simulink model "test_p"  (R2022a)
settings: Solver=FixedStepAuto  StartTime=0.0  StopTime=20  FixedStep=0.005  RelTol=1e-3
values from neighbouring files (symbols this model uses):
  AttDyna_Ixx = 0.0211    [InitParameters.m]
  AttDyna_Iyy = 0.0219    [InitParameters.m]
  AttDyna_Izz = 0.0366    [InitParameters.m]
  ConEfficiency_drone_cM = 1.779e-07    [InitParameters.m]
  ConEfficiency_drone_cT = 1.105e-05    [InitParameters.m]
  ConEfficiency_drone_R = 0.225    [InitParameters.m]
  PowerUnit_CR = 1148    [InitParameters.m]
  PowerUnit_Tm = 0.02    [InitParameters.m]
  PowerUnit_wb = -141.4    [InitParameters.m]
libraries: simulink x53, slpidlib x15, fuzblock x12, mpclib x1
(part 3 of 3)

== system test_p/四旋翼模型(简化)1/动力模型 ==
  In1 : Inport
  In2 : Inport  Port=2
  In3 : Inport  Port=3
  In4 : Inport  Port=4
  Constant{,1..3} (4 alike) : Constant  Value=1000
  Gain{,1..3} (4 alike) : Gain  Gain=1/1000
  Motor_Dynamics_1 : StateSpace  Commented=on  A=-1/PowerUnit_Tm  C=1/PowerUnit_Tm  D=0  InitialCondition=557.142*PowerUnit_Tm
  Motor_Dynamics_{2..5} (4 alike) : StateSpace  A=-1/PowerUnit_Tm  C=1/PowerUnit_Tm  D=0  InitialCondition=557.142*PowerUnit_Tm
  Mux : Mux
  Scope{,1..3} (4 alike) : Scope
  Subsystem : Subsystem
  Subsystem1 : Subsystem
  Subsystem2 : Subsystem
  Subsystem3 : Subsystem
  Sum{,1..3} (4 alike) : Sum  Inputs=|+-
  Transfer Fcn5 : TransferFcn  Commented=on  Denominator=[PowerUnit_Tm 1]
  Out1 : Outport  VectorParamsAs1DForOutWhenUnconnected=off
  wires:
  Subsystem2/1(Wss) -> Motor_Dynamics_4/1
  Mux/1 -> Out1/1
  Subsystem1/1(Wss) -> Motor_Dynamics_3/1
  Subsystem3/1(Wss) -> Motor_Dynamics_5/1
  Motor_Dynamics_2/1 -> Mux/1
  Motor_Dynamics_4/1 -> Mux/3
  Subsystem/1(Wss) -> Motor_Dynamics_2/1
  Motor_Dynamics_3/1 -> Mux/2
  Motor_Dynamics_5/1 -> Mux/4
  In1/1 -> Sum/1
  Sum/1 -> Scope3/1, Gain/1
  Gain/1 -> Subsystem/1("throttle_cmd ")
  Constant/1 -> Sum/2
  Constant1/1 -> Sum1/2
  Sum1/1 -> Scope2/1, Gain1/1
  In2/1 -> Sum1/1
  Gain1/1 -> Subsystem1/1("throttle_cmd ")
  In3/1 -> Sum2/1
  Sum2/1 -> Scope1/1, Gain2/1
  Constant2/1 -> Sum2/2
  Gain2/1 -> Subsystem2/1("throttle_cmd ")
  Constant3/1 -> Sum3/2
  Sum3/1 -> Scope/1, Gain3/1
  In4/1 -> Sum3/1
  Gain3/1 -> Subsystem3/1("throttle_cmd ")

== system test_p/四旋翼模型(简化)1/姿态动力学 ==
  note: Subsystem2
  t_x : Inport
  t_y : Inport  Port=2
  t_z : Inport  Port=3
  Constant1 : Constant  Value=AttDyna_Ixx
  Constant2 : Constant  Value=AttDyna_Izz
  Constant4 : Constant  Value=AttDyna_Iyy
  Integrator6 : Integrator
  Integrator7 : Integrator
  Integrator8 : Integrator
  Mux : Mux  Inputs=3
  att_dyna : MATLAB Function  TreatAsAtomicUnit=on
  wb_vector : Outport  VectorParamsAs1DForOutWhenUnconnected=off
  wbx : Outport  Port=2  VectorParamsAs1DForOutWhenUnconnected=off
  wby : Outport  Port=3  VectorParamsAs1DForOutWhenUnconnected=off
  wbz : Outport  Port=4  VectorParamsAs1DForOutWhenUnconnected=off
  wires:
  att_dyna/3(wbz_d) -> Integrator8/1
  att_dyna/2(wby_d) -> Integrator7/1
  att_dyna/1(wbx_d) -> Integrator6/1
  t_y/1 -> att_dyna/5(t_y)
  t_z/1 -> att_dyna/6(t_z)
  t_x/1 -> att_dyna/4(t_x)
  Integrator8/1 -> Mux/3, wbz/1
  Integrator6/1 -> Mux/1, wbx/1
  Integrator7/1 -> Mux/2, wby/1
  Constant2/1 -> att_dyna/3(Izz)
  Constant4/1 -> att_dyna/2(Iyy)
  Constant1/1 -> att_dyna/1(Ixx)
  Mux/1 -> wb_vector/1

== system test_p/四旋翼模型(简化)1/姿态运动学 ==
  pitch : Inport
  roll : Inport  Port=2
  wbx : Inport  Port=3
  wby : Inport  Port=4
  wbz : Inport  Port=5
  Integrator10 : Integrator
  Integrator11 : Integrator
  Integrator9 : Integrator
  att_kine : MATLAB Function  TreatAsAtomicUnit=on
  pitch_ : Outport  VectorParamsAs1DForOutWhenUnconnected=off
  roll_ : Outport  Port=2  VectorParamsAs1DForOutWhenUnconnected=off
  yaw : Outport  Port=3  VectorParamsAs1DForOutWhenUnconnected=off
  wires:
  Integrator9/1 -> roll_/1
  att_kine/1(roll_dot) -> Integrator9/1
  att_kine/2(pitch_dot) -> Integrator10/1
  Integrator11/1 -> yaw/1
  Integrator10/1 -> pitch_/1
  att_kine/3(yaw_dot) -> Integrator11/1
  roll/1 -> att_kine/5(roll)
  pitch/1 -> att_kine/4(pitch)
  wbx/1 -> att_kine/1(wbx)
  wby/1 -> att_kine/2(wby)
  wbz/1 -> att_kine/3(wbz)

== system test_p/四旋翼模型(简化)1/控制效率模型 ==
  w1 : Inport
  w2 : Inport  Port=2
  w3 : Inport  Port=3
  w4 : Inport  Port=4
  Constant5 : Constant  Value=ConEfficiency_drone_R
  Constant6 : Constant  Value=ConEfficiency_drone_cT
  Constant8 : Constant  Value=ConEfficiency_drone_cM
  control_efficiency : MATLAB Function  TreatAsAtomicUnit=on
  f : Outport  VectorParamsAs1DForOutWhenUnconnected=off
  t_x : Outport  Port=2  VectorParamsAs1DForOutWhenUnconnected=off
  t_y : Outport  Port=3  VectorParamsAs1DForOutWhenUnconnected=off
  t_z : Outport  Port=4  VectorParamsAs1DForOutWhenUnconnected=off
  wires:
  control_efficiency/1(f) -> f/1
  control_efficiency/4(t_z) -> t_z/1
  w4/1 -> control_efficiency/4(w4)
  control_efficiency/2(t_x) -> t_x/1
  w3/1 -> control_efficiency/3(w3)
  control_efficiency/3(t_y) -> t_y/1
  w2/1 -> control_efficiency/2(w2)
  Constant8/1 -> control_efficiency/7(cm)
  w1/1 -> control_efficiency/1(w1)
  Constant5/1 -> control_efficiency/5(d)
  Constant6/1 -> control_efficiency/6(ct)

== system test_p/四旋翼模型(简化)2/Control efficiency model ==
  w1 : Inport
  w2 : Inport  Port=2
  w3 : Inport  Port=3
  w4 : Inport  Port=4
  Constant5 : Constant  Value=ConEfficiency_drone_R
  Constant6 : Constant  Value=ConEfficiency_drone_cT
  Constant8 : Constant  Value=ConEfficiency_drone_cM
  control_efficiency : MATLAB Function  TreatAsAtomicUnit=on
  f : Outport  VectorParamsAs1DForOutWhenUnconnected=off
  t_x : Outport  Port=2  VectorParamsAs1DForOutWhenUnconnected=off
  t_y : Outport  Port=3  VectorParamsAs1DForOutWhenUnconnected=off
  t_z : Outport  Port=4  VectorParamsAs1DForOutWhenUnconnected=off
  wires:
  control_efficiency/1(f) -> f/1
  control_efficiency/4(t_z) -> t_z/1
  w4/1 -> control_efficiency/4(w4)
  control_efficiency/2(t_x) -> t_x/1
  w3/1 -> control_efficiency/3(w3)
  control_efficiency/3(t_y) -> t_y/1
  w2/1 -> control_efficiency/2(w2)
  Constant8/1 -> control_efficiency/7(cm)
  w1/1 -> control_efficiency/1(w1)
  Constant5/1 -> control_efficiency/5(d)
  Constant6/1 -> control_efficiency/6(ct)

== system test_p/四旋翼模型(简化)2/Kinetic model ==
  In1 : Inport
  In2 : Inport  Port=2
  In3 : Inport  Port=3
  In4 : Inport  Port=4
  Constant{,1..3} (4 alike) : Constant  Value=1000
  Gain{,1..3} (4 alike) : Gain  Gain=1/1000
  Motor_Dynamics_1 : StateSpace  Commented=on  A=-1/PowerUnit_Tm  C=1/PowerUnit_Tm  D=0  InitialCondition=557.142*PowerUnit_Tm
  Motor_Dynamics_{2..5} (4 alike) : StateSpace  A=-1/PowerUnit_Tm  C=1/PowerUnit_Tm  D=0  InitialCondition=557.142*PowerUnit_Tm
  Mux : Mux
  Scope{,1..3} (4 alike) : Scope
  Subsystem : Subsystem
  Subsystem1 : Subsystem
  Subsystem2 : Subsystem
  Subsystem3 : Subsystem
  Sum{,1..3} (4 alike) : Sum  Inputs=|+-
  Transfer Fcn5 : TransferFcn  Commented=on  Denominator=[PowerUnit_Tm 1]
  Out1 : Outport  VectorParamsAs1DForOutWhenUnconnected=off
  wires:
  Subsystem2/1(Wss) -> Motor_Dynamics_4/1
  Mux/1 -> Out1/1
  Subsystem1/1(Wss) -> Motor_Dynamics_3/1
  Subsystem3/1(Wss) -> Motor_Dynamics_5/1
  Motor_Dynamics_2/1 -> Mux/1
  Motor_Dynamics_4/1 -> Mux/3
  Subsystem/1(Wss) -> Motor_Dynamics_2/1
  Motor_Dynamics_3/1 -> Mux/2
  Motor_Dynamics_5/1 -> Mux/4
  In1/1 -> Sum/1
  Sum/1 -> Scope3/1, Gain/1
  Gain/1 -> Subsystem/1("throttle_cmd ")
  Constant/1 -> Sum/2
  Constant1/1 -> Sum1/2
  Sum1/1 -> Scope2/1, Gain1/1
  In2/1 -> Sum1/1
  Gain1/1 -> Subsystem1/1("throttle_cmd ")
  In3/1 -> Sum2/1
  Sum2/1 -> Scope1/1, Gain2/1
  Constant2/1 -> Sum2/2
  Gain2/1 -> Subsystem2/1("throttle_cmd ")
  Constant3/1 -> Sum3/2
  Sum3/1 -> Scope/1, Gain3/1
  In4/1 -> Sum3/1
  Gain3/1 -> Subsystem3/1("throttle_cmd ")

== system test_p/四旋翼模型(简化)2/Posture Kinematics ==
  pitch : Inport
  roll : Inport  Port=2
  wbx : Inport  Port=3
  wby : Inport  Port=4
  wbz : Inport  Port=5
  Integrator10 : Integrator
  Integrator11 : Integrator
  Integrator9 : Integrator
  att_kine : MATLAB Function  TreatAsAtomicUnit=on
  pitch_ : Outport  VectorParamsAs1DForOutWhenUnconnected=off
  roll_ : Outport  Port=2  VectorParamsAs1DForOutWhenUnconnected=off
  yaw : Outport  Port=3  VectorParamsAs1DForOutWhenUnconnected=off
  wires:
  Integrator9/1 -> roll_/1
  att_kine/1(roll_dot) -> Integrator9/1
  att_kine/2(pitch_dot) -> Integrator10/1
  Integrator11/1 -> yaw/1
  Integrator10/1 -> pitch_/1
  att_kine/3(yaw_dot) -> Integrator11/1
  roll/1 -> att_kine/5(roll)
  pitch/1 -> att_kine/4(pitch)
  wbx/1 -> att_kine/1(wbx)
  wby/1 -> att_kine/2(wby)
  wbz/1 -> att_kine/3(wbz)

== system test_p/四旋翼模型(简化)2/Posture dynamics ==
  note: Subsystem2
  t_x : Inport
  t_y : Inport  Port=2
  t_z : Inport  Port=3
  Constant1 : Constant  Value=AttDyna_Ixx
  Constant2 : Constant  Value=AttDyna_Izz
  Constant4 : Constant  Value=AttDyna_Iyy
  Integrator6 : Integrator
  Integrator7 : Integrator
  Integrator8 : Integrator
  Mux : Mux  Inputs=3
  att_dyna : MATLAB Function  TreatAsAtomicUnit=on
  wb_vector : Outport  VectorParamsAs1DForOutWhenUnconnected=off
  wbx : Outport  Port=2  VectorParamsAs1DForOutWhenUnconnected=off
  wby : Outport  Port=3  VectorParamsAs1DForOutWhenUnconnected=off
  wbz : Outport  Port=4  VectorParamsAs1DForOutWhenUnconnected=off
  wires:
  att_dyna/3(wbz_d) -> Integrator8/1
  att_dyna/2(wby_d) -> Integrator7/1
  att_dyna/1(wbx_d) -> Integrator6/1
  t_y/1 -> att_dyna/5(t_y)
  t_z/1 -> att_dyna/6(t_z)
  t_x/1 -> att_dyna/4(t_x)
  Integrator8/1 -> Mux/3, wbz/1
  Integrator6/1 -> Mux/1, wbx/1
  Integrator7/1 -> Mux/2, wby/1
  Constant2/1 -> att_dyna/3(Izz)
  Constant4/1 -> att_dyna/2(Iyy)
  Constant1/1 -> att_dyna/1(Ixx)
  Mux/1 -> wb_vector/1

== system test_p/四旋翼模型(简化)3/动力模型 ==
  In1 : Inport
  In2 : Inport  Port=2
  In3 : Inport  Port=3
  In4 : Inport  Port=4
  Constant{,1..3} (4 alike) : Constant  Value=1000
  Gain{,1..3} (4 alike) : Gain  Gain=1/1000
  Motor_Dynamics_1 : StateSpace  Commented=on  A=-1/PowerUnit_Tm  C=1/PowerUnit_Tm  D=0  InitialCondition=557.142*PowerUnit_Tm
  Motor_Dynamics_{2..5} (4 alike) : StateSpace  A=-1/PowerUnit_Tm  C=1/PowerUnit_Tm  D=0  InitialCondition=557.142*PowerUnit_Tm
  Mux : Mux
  Scope{,1..3} (4 alike) : Scope
  Subsystem : Subsystem
  Subsystem1 : Subsystem
  Subsystem2 : Subsystem
  Subsystem3 : Subsystem
  Sum{,1..3} (4 alike) : Sum  Inputs=|+-
  Transfer Fcn5 : TransferFcn  Commented=on  Denominator=[PowerUnit_Tm 1]
  Out1 : Outport  VectorParamsAs1DForOutWhenUnconnected=off
  wires:
  Subsystem2/1(Wss) -> Motor_Dynamics_4/1
  Mux/1 -> Out1/1
  Subsystem1/1(Wss) -> Motor_Dynamics_3/1
  Subsystem3/1(Wss) -> Motor_Dynamics_5/1
  Motor_Dynamics_2/1 -> Mux/1
  Motor_Dynamics_4/1 -> Mux/3
  Subsystem/1(Wss) -> Motor_Dynamics_2/1
  Motor_Dynamics_3/1 -> Mux/2
  Motor_Dynamics_5/1 -> Mux/4
  In1/1 -> Sum/1
  Sum/1 -> Scope3/1, Gain/1
  Gain/1 -> Subsystem/1("throttle_cmd ")
  Constant/1 -> Sum/2
  Constant1/1 -> Sum1/2
  Sum1/1 -> Scope2/1, Gain1/1
  In2/1 -> Sum1/1
  Gain1/1 -> Subsystem1/1("throttle_cmd ")
  In3/1 -> Sum2/1
  Sum2/1 -> Scope1/1, Gain2/1
  Constant2/1 -> Sum2/2
  Gain2/1 -> Subsystem2/1("throttle_cmd ")
  Constant3/1 -> Sum3/2
  Sum3/1 -> Scope/1, Gain3/1
  In4/1 -> Sum3/1
  Gain3/1 -> Subsystem3/1("throttle_cmd ")

== system test_p/四旋翼模型(简化)3/姿态动力学 ==
  note: Subsystem2
  t_x : Inport
  t_y : Inport  Port=2
  t_z : Inport  Port=3
  Constant1 : Constant  Value=AttDyna_Ixx
  Constant2 : Constant  Value=AttDyna_Izz
  Constant4 : Constant  Value=AttDyna_Iyy
  Integrator6 : Integrator
  Integrator7 : Integrator
  Integrator8 : Integrator
  Mux : Mux  Inputs=3
  att_dyna : MATLAB Function  TreatAsAtomicUnit=on
  wb_vector : Outport  VectorParamsAs1DForOutWhenUnconnected=off
  wbx : Outport  Port=2  VectorParamsAs1DForOutWhenUnconnected=off
  wby : Outport  Port=3  VectorParamsAs1DForOutWhenUnconnected=off
  wbz : Outport  Port=4  VectorParamsAs1DForOutWhenUnconnected=off
  wires:
  att_dyna/3(wbz_d) -> Integrator8/1
  att_dyna/2(wby_d) -> Integrator7/1
  att_dyna/1(wbx_d) -> Integrator6/1
  t_y/1 -> att_dyna/5(t_y)
  t_z/1 -> att_dyna/6(t_z)
  t_x/1 -> att_dyna/4(t_x)
  Integrator8/1 -> Mux/3, wbz/1
  Integrator6/1 -> Mux/1, wbx/1
  Integrator7/1 -> Mux/2, wby/1
  Constant2/1 -> att_dyna/3(Izz)
  Constant4/1 -> att_dyna/2(Iyy)
  Constant1/1 -> att_dyna/1(Ixx)
  Mux/1 -> wb_vector/1

== system test_p/四旋翼模型(简化)3/姿态运动学 ==
  pitch : Inport
  roll : Inport  Port=2
  wbx : Inport  Port=3
  wby : Inport  Port=4
  wbz : Inport  Port=5
  Integrator10 : Integrator
  Integrator11 : Integrator
  Integrator9 : Integrator
  att_kine : MATLAB Function  TreatAsAtomicUnit=on
  pitch_ : Outport  VectorParamsAs1DForOutWhenUnconnected=off
  roll_ : Outport  Port=2  VectorParamsAs1DForOutWhenUnconnected=off
  yaw : Outport  Port=3  VectorParamsAs1DForOutWhenUnconnected=off
  wires:
  Integrator9/1 -> roll_/1
  att_kine/1(roll_dot) -> Integrator9/1
  att_kine/2(pitch_dot) -> Integrator10/1
  Integrator11/1 -> yaw/1
  Integrator10/1 -> pitch_/1
  att_kine/3(yaw_dot) -> Integrator11/1
  roll/1 -> att_kine/5(roll)
  pitch/1 -> att_kine/4(pitch)
  wbx/1 -> att_kine/1(wbx)
  wby/1 -> att_kine/2(wby)
  wbz/1 -> att_kine/3(wbz)

== system test_p/四旋翼模型(简化)3/控制效率模型 ==
  w1 : Inport
  w2 : Inport  Port=2
  w3 : Inport  Port=3
  w4 : Inport  Port=4
  Constant5 : Constant  Value=ConEfficiency_drone_R
  Constant6 : Constant  Value=ConEfficiency_drone_cT
  Constant8 : Constant  Value=ConEfficiency_drone_cM
  control_efficiency : MATLAB Function  TreatAsAtomicUnit=on
  f : Outport  VectorParamsAs1DForOutWhenUnconnected=off
  t_x : Outport  Port=2  VectorParamsAs1DForOutWhenUnconnected=off
  t_y : Outport  Port=3  VectorParamsAs1DForOutWhenUnconnected=off
  t_z : Outport  Port=4  VectorParamsAs1DForOutWhenUnconnected=off
  wires:
  control_efficiency/1(f) -> f/1
  control_efficiency/4(t_z) -> t_z/1
  w4/1 -> control_efficiency/4(w4)
  control_efficiency/2(t_x) -> t_x/1
  w3/1 -> control_efficiency/3(w3)
  control_efficiency/3(t_y) -> t_y/1
  w2/1 -> control_efficiency/2(w2)
  Constant8/1 -> control_efficiency/7(cm)
  w1/1 -> control_efficiency/1(w1)
  Constant5/1 -> control_efficiency/5(d)
  Constant6/1 -> control_efficiency/6(ct)

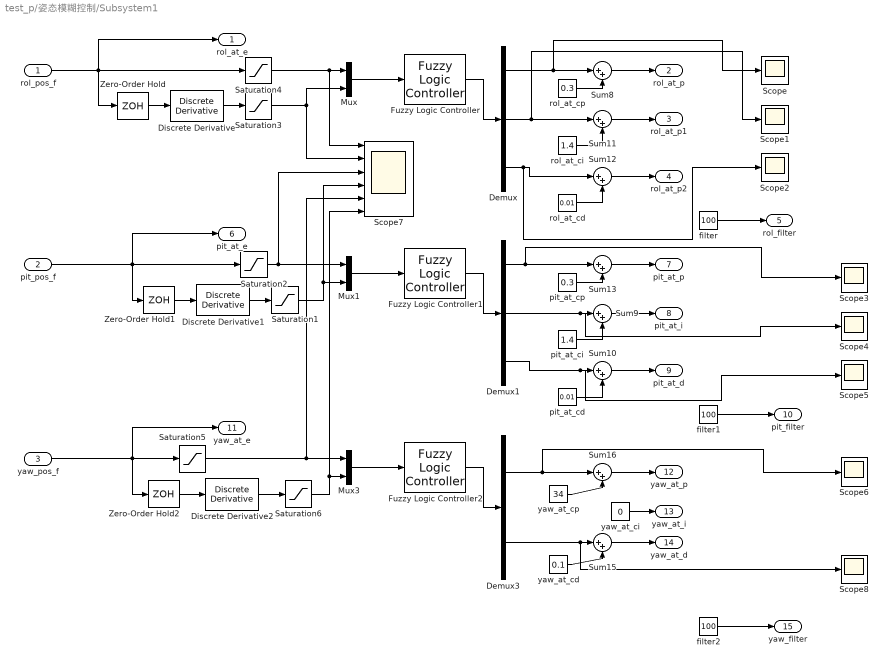
== system test_p/姿态模糊控制/Subsystem1 ==
  rol_pos_f : Inport
  pit_pos_f : Inport  Port=2
  yaw_pos_f : Inport  Port=3
  Demux : Demux  Outputs=3
  Demux1 : Demux  Outputs=3
  Demux3 : Demux  Outputs=2
  Discrete Derivative : simulink/Discrete/Discrete Derivative  gainval=1.0  ICPrevScaledInput=0.0  OutMin=[]  OutMax=[]  OutDataType=fixdt(1, 16)  OutScaling=2^-10  DoSatur=off
  Discrete Derivative1 : simulink/Discrete/Discrete Derivative  gainval=1.0  ICPrevScaledInput=0.0  OutMin=[]  OutMax=[]  OutDataType=fixdt(1, 16)  OutScaling=2^-10  DoSatur=off
  Discrete Derivative2 : simulink/Discrete/Discrete Derivative  gainval=1.0  ICPrevScaledInput=0.0  OutMin=[]  OutMax=[]  OutDataType=fixdt(1, 16)  OutScaling=2^-10  DoSatur=off
  Fuzzy Logic Controller : fuzblock/Fuzzy Logic  Controller  FIS='rol_pit_at.fis'  OutputSampleNumber=101  DataType=double  FuzzifiedInputs=off  RuleFiringStrengths=off  RuleOutputs=off  AggregatedOutputs=off  SimulateUsing=Interpreted execution  OutOfRangeInputValueMessage=warning  NoRuleFiredMessage=warning  EmptyOutputFuzzySetMessage=warning
  Fuzzy Logic Controller1 : fuzblock/Fuzzy Logic  Controller  FIS='rol_pit_at.fis'  OutputSampleNumber=101  DataType=double  FuzzifiedInputs=off  RuleFiringStrengths=off  RuleOutputs=off  AggregatedOutputs=off  SimulateUsing=Interpreted execution  OutOfRangeInputValueMessage=warning  NoRuleFiredMessage=warning  EmptyOutputFuzzySetMessage=warning
  Fuzzy Logic Controller2 : fuzblock/Fuzzy Logic  Controller  FIS='yaw_at.fis'  OutputSampleNumber=101  DataType=double  FuzzifiedInputs=off  RuleFiringStrengths=off  RuleOutputs=off  AggregatedOutputs=off  SimulateUsing=Interpreted execution  OutOfRangeInputValueMessage=warning  NoRuleFiredMessage=warning  EmptyOutputFuzzySetMessage=warning
  Mux : Mux  Inputs=2
  Mux1 : Mux  Inputs=2
  Mux3 : Mux  Inputs=2
  Saturation{1..6} (6 alike) : Saturate  UpperLimit=10  LowerLimit=-10
  Scope{,1..6,8} (8 alike) : Scope
  Scope7 : Scope  NumInputPorts=6
  Sum{8..13,15..16} (8 alike) : Sum  Inputs=|++
  Zero-Order Hold : ZeroOrderHold  SampleTime=-1
  Zero-Order Hold1 : ZeroOrderHold  SampleTime=-1
  Zero-Order Hold2 : ZeroOrderHold  SampleTime=-1
  filter : Constant  Value=100
  filter1 : Constant  Value=100
  filter2 : Constant  Value=100
  pit_at_cd : Constant  Value=0.01
  pit_at_ci : Constant  Value=1.4
  pit_at_cp : Constant  Value=0.3
  rol_at_cd : Constant  Value=0.01
  rol_at_ci : Constant  Value=1.4
  rol_at_cp : Constant  Value=0.3
  yaw_at_cd : Constant  Value=0.1
  yaw_at_ci : Constant  Value=0
  yaw_at_cp : Constant  Value=34
  rol_at_e : Outport  VectorParamsAs1DForOutWhenUnconnected=off
  rol_at_p : Outport  Port=2  VectorParamsAs1DForOutWhenUnconnected=off
  rol_at_p1 : Outport  Port=3  VectorParamsAs1DForOutWhenUnconnected=off
  rol_at_p2 : Outport  Port=4  VectorParamsAs1DForOutWhenUnconnected=off
  rol_filter : Outport  Port=5  VectorParamsAs1DForOutWhenUnconnected=off
  pit_at_e : Outport  Port=6  VectorParamsAs1DForOutWhenUnconnected=off
  pit_at_p : Outport  Port=7  VectorParamsAs1DForOutWhenUnconnected=off
  pit_at_i : Outport  Port=8  VectorParamsAs1DForOutWhenUnconnected=off
  pit_at_d : Outport  Port=9  VectorParamsAs1DForOutWhenUnconnected=off
  pit_filter : Outport  Port=10  VectorParamsAs1DForOutWhenUnconnected=off
  yaw_at_e : Outport  Port=11  VectorParamsAs1DForOutWhenUnconnected=off
  yaw_at_p : Outport  Port=12  VectorParamsAs1DForOutWhenUnconnected=off
  yaw_at_i : Outport  Port=13  VectorParamsAs1DForOutWhenUnconnected=off
  yaw_at_d : Outport  Port=14  VectorParamsAs1DForOutWhenUnconnected=off
  yaw_filter : Outport  Port=15  VectorParamsAs1DForOutWhenUnconnected=off
  wires:
  Discrete Derivative/1 -> Saturation3/1
  rol_at_ci/1 -> Sum11/2
  Mux3/1 -> Fuzzy Logic Controller2/1
  rol_pos_f/1 -> rol_at_e/1, Zero-Order Hold/1, Saturation4/1
  Demux/1 -> Scope/1, Sum8/1
  Zero-Order Hold2/1 -> Discrete Derivative2/1
  Sum12/1 -> rol_at_p2/1
  Demux1/2 -> Scope4/1, Sum9/1
  yaw_at_cp/1 -> Sum16/2
  yaw_pos_f/1 -> yaw_at_e/1, Zero-Order Hold2/1, Saturation5/1
  Sum11/1 -> rol_at_p1/1
  Discrete Derivative2/1 -> Saturation6/1
  Sum9/1 -> pit_at_i/1
  Mux1/1 -> Fuzzy Logic Controller1/1
  Sum13/1 -> pit_at_p/1
  Demux/3 -> Scope2/1, Sum12/1
  Sum8/1 -> rol_at_p/1
  Demux1/1 -> Scope3/1, Sum13/1
  yaw_at_cd/1 -> Sum15/2
  Zero-Order Hold1/1 -> Discrete Derivative1/1
  Zero-Order Hold/1 -> Discrete Derivative/1
  Demux3/1 -> Scope6/1, Sum16/1
  rol_at_cp/1 -> Sum8/2
  Fuzzy Logic Controller2/1 -> Demux3/1
  Sum16/1 -> yaw_at_p/1
  Sum15/1 -> yaw_at_d/1
  rol_at_cd/1 -> Sum12/2
  pit_pos_f/1 -> pit_at_e/1, Zero-Order Hold1/1, Saturation2/1
  Fuzzy Logic Controller1/1 -> Demux1/1
  Fuzzy Logic Controller/1 -> Demux/1
  pit_at_cp/1 -> Sum13/2
  Demux/2 -> Scope1/1, Sum11/1
  Mux/1 -> Fuzzy Logic Controller/1
  pit_at_ci/1 -> Sum9/2
  Sum10/1 -> pit_at_d/1
  Demux1/3 -> Scope5/1, Sum10/1
  pit_at_cd/1 -> Sum10/2
  filter/1 -> rol_filter/1
  filter1/1 -> pit_filter/1
  filter2/1 -> yaw_filter/1
  yaw_at_ci/1 -> yaw_at_i/1
  Demux3/2 -> Scope8/1, Sum15/1
  Discrete Derivative1/1 -> Saturation1/1
  Saturation1/1 -> Scope7/4, Mux1/2
  Saturation2/1 -> Scope7/3, Mux1/1
  Saturation3/1 -> Scope7/2, Mux/2
  Saturation4/1 -> Scope7/1, Mux/1
  Saturation5/1 -> Scope7/5, Mux3/1
  Saturation6/1 -> Scope7/6, Mux3/2

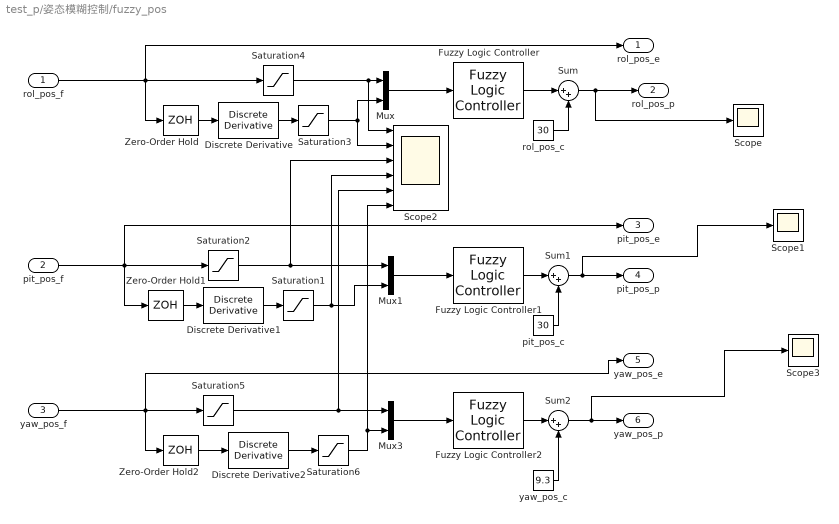
== system test_p/姿态模糊控制/fuzzy_pos ==
  rol_pos_f : Inport
  pit_pos_f : Inport  Port=2
  yaw_pos_f : Inport  Port=3
  Discrete Derivative : simulink/Discrete/Discrete Derivative  gainval=1.0  ICPrevScaledInput=0.0  OutMin=[]  OutMax=[]  OutDataType=fixdt(1, 16)  OutScaling=2^-10  DoSatur=off
  Discrete Derivative1 : simulink/Discrete/Discrete Derivative  gainval=1.0  ICPrevScaledInput=0.0  OutMin=[]  OutMax=[]  OutDataType=fixdt(1, 16)  OutScaling=2^-10  DoSatur=off
  Discrete Derivative2 : simulink/Discrete/Discrete Derivative  gainval=1.0  ICPrevScaledInput=0.0  OutMin=[]  OutMax=[]  OutDataType=fixdt(1, 16)  OutScaling=2^-10  DoSatur=off
  Fuzzy Logic Controller : fuzblock/Fuzzy Logic  Controller  FIS='rol_pit_pos.fis'  OutputSampleNumber=101  DataType=double  FuzzifiedInputs=off  RuleFiringStrengths=off  RuleOutputs=off  AggregatedOutputs=off  SimulateUsing=Interpreted execution  OutOfRangeInputValueMessage=warning  NoRuleFiredMessage=warning  EmptyOutputFuzzySetMessage=warning
  Fuzzy Logic Controller1 : fuzblock/Fuzzy Logic  Controller  FIS='rol_pit_pos.fis'  OutputSampleNumber=101  DataType=double  FuzzifiedInputs=off  RuleFiringStrengths=off  RuleOutputs=off  AggregatedOutputs=off  SimulateUsing=Interpreted execution  OutOfRangeInputValueMessage=warning  NoRuleFiredMessage=warning  EmptyOutputFuzzySetMessage=warning
  Fuzzy Logic Controller2 : fuzblock/Fuzzy Logic  Controller  FIS='yaw_pos.fis'  OutputSampleNumber=101  DataType=double  FuzzifiedInputs=off  RuleFiringStrengths=off  RuleOutputs=off  AggregatedOutputs=off  SimulateUsing=Interpreted execution  OutOfRangeInputValueMessage=warning  NoRuleFiredMessage=warning  EmptyOutputFuzzySetMessage=warning
  Mux : Mux  Inputs=2
  Mux1 : Mux  Inputs=2
  Mux3 : Mux  Inputs=2
  Saturation{1..6} (6 alike) : Saturate  UpperLimit=10  LowerLimit=-10
  Scope : Scope
  Scope1 : Scope
  Scope2 : Scope  NumInputPorts=6
  Scope3 : Scope
  Sum : Sum  Inputs=|++
  Sum1 : Sum  Inputs=|++
  Sum2 : Sum  Inputs=|++
  Zero-Order Hold : ZeroOrderHold  SampleTime=-1
  Zero-Order Hold1 : ZeroOrderHold  SampleTime=-1
  Zero-Order Hold2 : ZeroOrderHold  SampleTime=-1
  pit_pos_c : Constant  Value=30
  rol_pos_c : Constant  Value=30
  yaw_pos_c : Constant  Value=9.3
  rol_pos_e : Outport  VectorParamsAs1DForOutWhenUnconnected=off
  rol_pos_p : Outport  Port=2  VectorParamsAs1DForOutWhenUnconnected=off
  pit_pos_e : Outport  Port=3  VectorParamsAs1DForOutWhenUnconnected=off
  pit_pos_p : Outport  Port=4  VectorParamsAs1DForOutWhenUnconnected=off
  yaw_pos_e : Outport  Port=5  VectorParamsAs1DForOutWhenUnconnected=off
  yaw_pos_p : Outport  Port=6  VectorParamsAs1DForOutWhenUnconnected=off
  wires:
  Zero-Order Hold2/1 -> Discrete Derivative2/1
  pit_pos_f/1 -> pit_pos_e/1, Saturation2/1, Zero-Order Hold1/1
  rol_pos_f/1 -> rol_pos_e/1, Zero-Order Hold/1, Saturation4/1
  yaw_pos_f/1 -> yaw_pos_e/1, Zero-Order Hold2/1, Saturation5/1
  Discrete Derivative/1 -> Saturation3/1
  Mux3/1 -> Fuzzy Logic Controller2/1
  Zero-Order Hold1/1 -> Discrete Derivative1/1
  Mux1/1 -> Fuzzy Logic Controller1/1
  Mux/1 -> Fuzzy Logic Controller/1
  Zero-Order Hold/1 -> Discrete Derivative/1
  Discrete Derivative2/1 -> Saturation6/1
  Fuzzy Logic Controller/1 -> Sum/1
  Sum/1 -> Scope/1, rol_pos_p/1
  rol_pos_c/1 -> Sum/2
  Fuzzy Logic Controller1/1 -> Sum1/1
  pit_pos_c/1 -> Sum1/2
  Sum1/1 -> Scope1/1, pit_pos_p/1
  Fuzzy Logic Controller2/1 -> Sum2/1
  Sum2/1 -> Scope3/1, yaw_pos_p/1
  yaw_pos_c/1 -> Sum2/2
  Discrete Derivative1/1 -> Saturation1/1
  Saturation1/1 -> Scope2/4, Mux1/2
  Saturation2/1 -> Scope2/3, Mux1/1
  Saturation3/1 -> Mux/2, Scope2/2
  Saturation4/1 -> Scope2/1, Mux/1
  Saturation5/1 -> Scope2/5, Mux3/1
  Saturation6/1 -> Scope2/6, Mux3/2

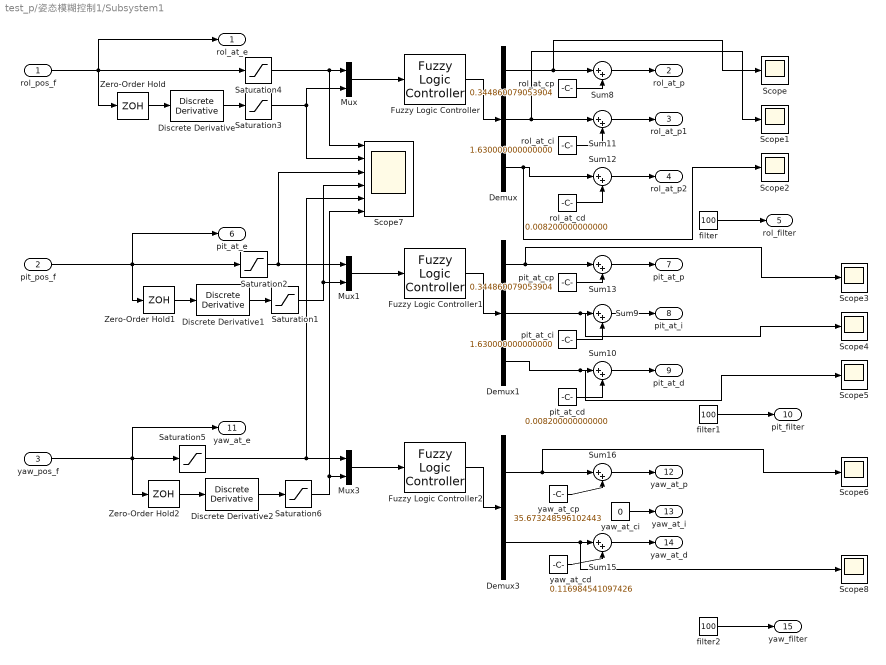
== system test_p/姿态模糊控制1/Subsystem1 ==
  rol_pos_f : Inport
  pit_pos_f : Inport  Port=2
  yaw_pos_f : Inport  Port=3
  Demux : Demux  Outputs=3
  Demux1 : Demux  Outputs=3
  Demux3 : Demux  Outputs=2
  Discrete Derivative : simulink/Discrete/Discrete Derivative  gainval=1.0  ICPrevScaledInput=0.0  OutMin=[]  OutMax=[]  OutDataType=fixdt(1, 16)  OutScaling=2^-10  DoSatur=off
  Discrete Derivative1 : simulink/Discrete/Discrete Derivative  gainval=1.0  ICPrevScaledInput=0.0  OutMin=[]  OutMax=[]  OutDataType=fixdt(1, 16)  OutScaling=2^-10  DoSatur=off
  Discrete Derivative2 : simulink/Discrete/Discrete Derivative  gainval=1.0  ICPrevScaledInput=0.0  OutMin=[]  OutMax=[]  OutDataType=fixdt(1, 16)  OutScaling=2^-10  DoSatur=off
  Fuzzy Logic Controller : fuzblock/Fuzzy Logic  Controller  FIS='rol_pit_at.fis'  OutputSampleNumber=101  DataType=double  FuzzifiedInputs=off  RuleFiringStrengths=off  RuleOutputs=off  AggregatedOutputs=off  SimulateUsing=Interpreted execution  OutOfRangeInputValueMessage=warning  NoRuleFiredMessage=warning  EmptyOutputFuzzySetMessage=warning
  Fuzzy Logic Controller1 : fuzblock/Fuzzy Logic  Controller  FIS='rol_pit_at.fis'  OutputSampleNumber=101  DataType=double  FuzzifiedInputs=off  RuleFiringStrengths=off  RuleOutputs=off  AggregatedOutputs=off  SimulateUsing=Interpreted execution  OutOfRangeInputValueMessage=warning  NoRuleFiredMessage=warning  EmptyOutputFuzzySetMessage=warning
  Fuzzy Logic Controller2 : fuzblock/Fuzzy Logic  Controller  FIS='yaw_at.fis'  OutputSampleNumber=101  DataType=double  FuzzifiedInputs=off  RuleFiringStrengths=off  RuleOutputs=off  AggregatedOutputs=off  SimulateUsing=Interpreted execution  OutOfRangeInputValueMessage=warning  NoRuleFiredMessage=warning  EmptyOutputFuzzySetMessage=warning
  Mux : Mux  Inputs=2
  Mux1 : Mux  Inputs=2
  Mux3 : Mux  Inputs=2
  Saturation{1..6} (6 alike) : Saturate  UpperLimit=10  LowerLimit=-10
  Scope{,1..6,8} (8 alike) : Scope
  Scope7 : Scope  NumInputPorts=6
  Sum{8..13,15..16} (8 alike) : Sum  Inputs=|++
  Zero-Order Hold : ZeroOrderHold  SampleTime=-1
  Zero-Order Hold1 : ZeroOrderHold  SampleTime=-1
  Zero-Order Hold2 : ZeroOrderHold  SampleTime=-1
  filter : Constant  Value=100
  filter1 : Constant  Value=100
  filter2 : Constant  Value=100
  pit_at_cd : Constant  Value=0.008200000000000
  pit_at_ci : Constant  Value=1.630000000000000
  pit_at_cp : Constant  Value=0.344860079053904
  rol_at_cd : Constant  Value=0.008200000000000
  rol_at_ci : Constant  Value=1.630000000000000
  rol_at_cp : Constant  Value=0.344860079053904
  yaw_at_cd : Constant  Value=0.116984541097426
  yaw_at_ci : Constant  Value=0
  yaw_at_cp : Constant  Value=35.673248596102443
  rol_at_e : Outport  VectorParamsAs1DForOutWhenUnconnected=off
  rol_at_p : Outport  Port=2  VectorParamsAs1DForOutWhenUnconnected=off
  rol_at_p1 : Outport  Port=3  VectorParamsAs1DForOutWhenUnconnected=off
  rol_at_p2 : Outport  Port=4  VectorParamsAs1DForOutWhenUnconnected=off
  rol_filter : Outport  Port=5  VectorParamsAs1DForOutWhenUnconnected=off
  pit_at_e : Outport  Port=6  VectorParamsAs1DForOutWhenUnconnected=off
  pit_at_p : Outport  Port=7  VectorParamsAs1DForOutWhenUnconnected=off
  pit_at_i : Outport  Port=8  VectorParamsAs1DForOutWhenUnconnected=off
  pit_at_d : Outport  Port=9  VectorParamsAs1DForOutWhenUnconnected=off
  pit_filter : Outport  Port=10  VectorParamsAs1DForOutWhenUnconnected=off
  yaw_at_e : Outport  Port=11  VectorParamsAs1DForOutWhenUnconnected=off
  yaw_at_p : Outport  Port=12  VectorParamsAs1DForOutWhenUnconnected=off
  yaw_at_i : Outport  Port=13  VectorParamsAs1DForOutWhenUnconnected=off
  yaw_at_d : Outport  Port=14  VectorParamsAs1DForOutWhenUnconnected=off
  yaw_filter : Outport  Port=15  VectorParamsAs1DForOutWhenUnconnected=off
  wires:
  Discrete Derivative/1 -> Saturation3/1
  rol_at_ci/1 -> Sum11/2
  Mux3/1 -> Fuzzy Logic Controller2/1
  rol_pos_f/1 -> rol_at_e/1, Zero-Order Hold/1, Saturation4/1
  Demux/1 -> Scope/1, Sum8/1
  Zero-Order Hold2/1 -> Discrete Derivative2/1
  Sum12/1 -> rol_at_p2/1
  Demux1/2 -> Scope4/1, Sum9/1
  yaw_at_cp/1 -> Sum16/2
  yaw_pos_f/1 -> yaw_at_e/1, Zero-Order Hold2/1, Saturation5/1
  Sum11/1 -> rol_at_p1/1
  Discrete Derivative2/1 -> Saturation6/1
  Sum9/1 -> pit_at_i/1
  Mux1/1 -> Fuzzy Logic Controller1/1
  Sum13/1 -> pit_at_p/1
  Demux/3 -> Scope2/1, Sum12/1
  Sum8/1 -> rol_at_p/1
  Demux1/1 -> Scope3/1, Sum13/1
  yaw_at_cd/1 -> Sum15/2
  Zero-Order Hold1/1 -> Discrete Derivative1/1
  Zero-Order Hold/1 -> Discrete Derivative/1
  Demux3/1 -> Scope6/1, Sum16/1
  rol_at_cp/1 -> Sum8/2
  Fuzzy Logic Controller2/1 -> Demux3/1
  Sum16/1 -> yaw_at_p/1
  Sum15/1 -> yaw_at_d/1
  rol_at_cd/1 -> Sum12/2
  pit_pos_f/1 -> pit_at_e/1, Zero-Order Hold1/1, Saturation2/1
  Fuzzy Logic Controller1/1 -> Demux1/1
  Fuzzy Logic Controller/1 -> Demux/1
  pit_at_cp/1 -> Sum13/2
  Demux/2 -> Scope1/1, Sum11/1
  Mux/1 -> Fuzzy Logic Controller/1
  pit_at_ci/1 -> Sum9/2
  Sum10/1 -> pit_at_d/1
  Demux1/3 -> Scope5/1, Sum10/1
  pit_at_cd/1 -> Sum10/2
  filter/1 -> rol_filter/1
  filter1/1 -> pit_filter/1
  filter2/1 -> yaw_filter/1
  yaw_at_ci/1 -> yaw_at_i/1
  Demux3/2 -> Scope8/1, Sum15/1
  Discrete Derivative1/1 -> Saturation1/1
  Saturation1/1 -> Scope7/4, Mux1/2
  Saturation2/1 -> Scope7/3, Mux1/1
  Saturation3/1 -> Scope7/2, Mux/2
  Saturation4/1 -> Scope7/1, Mux/1
  Saturation5/1 -> Scope7/5, Mux3/1
  Saturation6/1 -> Scope7/6, Mux3/2

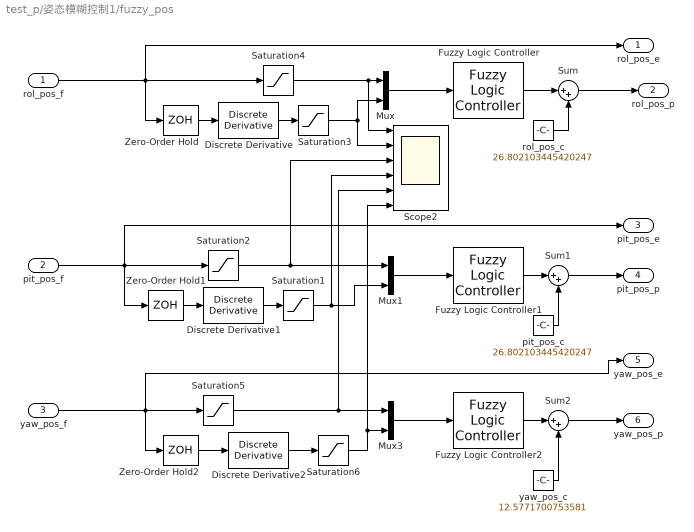
== system test_p/姿态模糊控制1/fuzzy_pos ==
  rol_pos_f : Inport
  pit_pos_f : Inport  Port=2
  yaw_pos_f : Inport  Port=3
  Discrete Derivative : simulink/Discrete/Discrete Derivative  gainval=1.0  ICPrevScaledInput=0.0  OutMin=[]  OutMax=[]  OutDataType=fixdt(1, 16)  OutScaling=2^-10  DoSatur=off
  Discrete Derivative1 : simulink/Discrete/Discrete Derivative  gainval=1.0  ICPrevScaledInput=0.0  OutMin=[]  OutMax=[]  OutDataType=fixdt(1, 16)  OutScaling=2^-10  DoSatur=off
  Discrete Derivative2 : simulink/Discrete/Discrete Derivative  gainval=1.0  ICPrevScaledInput=0.0  OutMin=[]  OutMax=[]  OutDataType=fixdt(1, 16)  OutScaling=2^-10  DoSatur=off
  Fuzzy Logic Controller : fuzblock/Fuzzy Logic  Controller  FIS='rol_pit_pos.fis'  OutputSampleNumber=101  DataType=double  FuzzifiedInputs=off  RuleFiringStrengths=off  RuleOutputs=off  AggregatedOutputs=off  SimulateUsing=Interpreted execution  OutOfRangeInputValueMessage=warning  NoRuleFiredMessage=warning  EmptyOutputFuzzySetMessage=warning
  Fuzzy Logic Controller1 : fuzblock/Fuzzy Logic  Controller  FIS='rol_pit_pos.fis'  OutputSampleNumber=101  DataType=double  FuzzifiedInputs=off  RuleFiringStrengths=off  RuleOutputs=off  AggregatedOutputs=off  SimulateUsing=Interpreted execution  OutOfRangeInputValueMessage=warning  NoRuleFiredMessage=warning  EmptyOutputFuzzySetMessage=warning
  Fuzzy Logic Controller2 : fuzblock/Fuzzy Logic  Controller  FIS='yaw_pos.fis'  OutputSampleNumber=101  DataType=double  FuzzifiedInputs=off  RuleFiringStrengths=off  RuleOutputs=off  AggregatedOutputs=off  SimulateUsing=Interpreted execution  OutOfRangeInputValueMessage=warning  NoRuleFiredMessage=warning  EmptyOutputFuzzySetMessage=warning
  Mux : Mux  Inputs=2
  Mux1 : Mux  Inputs=2
  Mux3 : Mux  Inputs=2
  Saturation{1..6} (6 alike) : Saturate  UpperLimit=10  LowerLimit=-10
  Scope2 : Scope  NumInputPorts=6
  Sum : Sum  Inputs=|++
  Sum1 : Sum  Inputs=|++
  Sum2 : Sum  Inputs=|++
  Zero-Order Hold : ZeroOrderHold  SampleTime=-1
  Zero-Order Hold1 : ZeroOrderHold  SampleTime=-1
  Zero-Order Hold2 : ZeroOrderHold  SampleTime=-1
  pit_pos_c : Constant  Value=26.802103445420247
  rol_pos_c : Constant  Value=26.802103445420247
  yaw_pos_c : Constant  Value=12.5771700753581
  rol_pos_e : Outport  VectorParamsAs1DForOutWhenUnconnected=off
  rol_pos_p : Outport  Port=2  VectorParamsAs1DForOutWhenUnconnected=off
  pit_pos_e : Outport  Port=3  VectorParamsAs1DForOutWhenUnconnected=off
  pit_pos_p : Outport  Port=4  VectorParamsAs1DForOutWhenUnconnected=off
  yaw_pos_e : Outport  Port=5  VectorParamsAs1DForOutWhenUnconnected=off
  yaw_pos_p : Outport  Port=6  VectorParamsAs1DForOutWhenUnconnected=off
  wires:
  Zero-Order Hold2/1 -> Discrete Derivative2/1
  pit_pos_f/1 -> pit_pos_e/1, Saturation2/1, Zero-Order Hold1/1
  rol_pos_f/1 -> rol_pos_e/1, Zero-Order Hold/1, Saturation4/1
  yaw_pos_f/1 -> yaw_pos_e/1, Zero-Order Hold2/1, Saturation5/1
  Discrete Derivative/1 -> Saturation3/1
  Mux3/1 -> Fuzzy Logic Controller2/1
  Zero-Order Hold1/1 -> Discrete Derivative1/1
  Mux1/1 -> Fuzzy Logic Controller1/1
  Mux/1 -> Fuzzy Logic Controller/1
  Zero-Order Hold/1 -> Discrete Derivative/1
  Discrete Derivative2/1 -> Saturation6/1
  Fuzzy Logic Controller/1 -> Sum/1
  Sum/1 -> rol_pos_p/1
  rol_pos_c/1 -> Sum/2
  Fuzzy Logic Controller1/1 -> Sum1/1
  pit_pos_c/1 -> Sum1/2
  Sum1/1 -> pit_pos_p/1
  Fuzzy Logic Controller2/1 -> Sum2/1
  Sum2/1 -> yaw_pos_p/1
  yaw_pos_c/1 -> Sum2/2
  Discrete Derivative1/1 -> Saturation1/1
  Saturation1/1 -> Scope2/4, Mux1/2
  Saturation2/1 -> Scope2/3, Mux1/1
  Saturation3/1 -> Mux/2, Scope2/2
  Saturation4/1 -> Scope2/1, Mux/1
  Saturation5/1 -> Scope2/5, Mux3/1
  Saturation6/1 -> Scope2/6, Mux3/2

== system test_p/四旋翼模型(简化)/动力模型/Subsystem ==
  "throttle_cmd " : Inport
  CR : Gain  Gain=PowerUnit_CR
  Sum : Sum  Inputs=|++
  wb(转速常参数) : Constant  Value=PowerUnit_wb
  Wss : Outport  VectorParamsAs1DForOutWhenUnconnected=off
  wires:
  "throttle_cmd "/1 -> CR/1
  CR/1 -> Sum/1
  wb(转速常参数)/1 -> Sum/2
  Sum/1 -> Wss/1  "Wss"

== system test_p/四旋翼模型(简化)/动力模型/Subsystem1 ==
  "throttle_cmd " : Inport
  CR : Gain  Gain=PowerUnit_CR
  Sum : Sum  Inputs=|++
  wb(转速常参数) : Constant  Value=PowerUnit_wb
  Wss : Outport  VectorParamsAs1DForOutWhenUnconnected=off
  wires:
  Sum/1 -> Wss/1  "Wss"
  wb(转速常参数)/1 -> Sum/2
  CR/1 -> Sum/1
  "throttle_cmd "/1 -> CR/1

== system test_p/四旋翼模型(简化)/动力模型/Subsystem2 ==
  "throttle_cmd " : Inport
  CR : Gain  Gain=PowerUnit_CR
  Sum : Sum  Inputs=|++
  wb(转速常参数) : Constant  Value=PowerUnit_wb
  Wss : Outport  VectorParamsAs1DForOutWhenUnconnected=off
  wires:
  "throttle_cmd "/1 -> CR/1
  CR/1 -> Sum/1
  wb(转速常参数)/1 -> Sum/2
  Sum/1 -> Wss/1  "Wss"

== system test_p/四旋翼模型(简化)/动力模型/Subsystem3 ==
  "throttle_cmd " : Inport
  CR : Gain  Gain=PowerUnit_CR
  Sum : Sum  Inputs=|++
  wb(转速常参数) : Constant  Value=PowerUnit_wb
  Wss : Outport  VectorParamsAs1DForOutWhenUnconnected=off
  wires:
  Sum/1 -> Wss/1  "Wss"
  wb(转速常参数)/1 -> Sum/2
  CR/1 -> Sum/1
  "throttle_cmd "/1 -> CR/1

== system test_p/四旋翼模型(简化)1/动力模型/Subsystem ==
  "throttle_cmd " : Inport
  CR : Gain  Gain=PowerUnit_CR
  Sum : Sum  Inputs=|++
  wb(转速常参数) : Constant  Value=PowerUnit_wb
  Wss : Outport  VectorParamsAs1DForOutWhenUnconnected=off
  wires:
  "throttle_cmd "/1 -> CR/1
  CR/1 -> Sum/1
  wb(转速常参数)/1 -> Sum/2
  Sum/1 -> Wss/1  "Wss"

== system test_p/四旋翼模型(简化)1/动力模型/Subsystem1 ==
  "throttle_cmd " : Inport
  CR : Gain  Gain=PowerUnit_CR
  Sum : Sum  Inputs=|++
  wb(转速常参数) : Constant  Value=PowerUnit_wb
  Wss : Outport  VectorParamsAs1DForOutWhenUnconnected=off
  wires:
  Sum/1 -> Wss/1  "Wss"
  wb(转速常参数)/1 -> Sum/2
  CR/1 -> Sum/1
  "throttle_cmd "/1 -> CR/1

== system test_p/四旋翼模型(简化)1/动力模型/Subsystem2 ==
  "throttle_cmd " : Inport
  CR : Gain  Gain=PowerUnit_CR
  Sum : Sum  Inputs=|++
  wb(转速常参数) : Constant  Value=PowerUnit_wb
  Wss : Outport  VectorParamsAs1DForOutWhenUnconnected=off
  wires:
  "throttle_cmd "/1 -> CR/1
  CR/1 -> Sum/1
  wb(转速常参数)/1 -> Sum/2
  Sum/1 -> Wss/1  "Wss"

== system test_p/四旋翼模型(简化)1/动力模型/Subsystem3 ==
  "throttle_cmd " : Inport
  CR : Gain  Gain=PowerUnit_CR
  Sum : Sum  Inputs=|++
  wb(转速常参数) : Constant  Value=PowerUnit_wb
  Wss : Outport  VectorParamsAs1DForOutWhenUnconnected=off
  wires:
  Sum/1 -> Wss/1  "Wss"
  wb(转速常参数)/1 -> Sum/2
  CR/1 -> Sum/1
  "throttle_cmd "/1 -> CR/1

== system test_p/四旋翼模型(简化)2/Kinetic model/Subsystem ==
  "throttle_cmd " : Inport
  CR : Gain  Gain=PowerUnit_CR
  Sum : Sum  Inputs=|++
  wb(转速常参数) : Constant  Value=PowerUnit_wb
  Wss : Outport  VectorParamsAs1DForOutWhenUnconnected=off
  wires:
  "throttle_cmd "/1 -> CR/1
  CR/1 -> Sum/1
  wb(转速常参数)/1 -> Sum/2
  Sum/1 -> Wss/1  "Wss"

== system test_p/四旋翼模型(简化)2/Kinetic model/Subsystem1 ==
  "throttle_cmd " : Inport
  CR : Gain  Gain=PowerUnit_CR
  Sum : Sum  Inputs=|++
  wb(转速常参数) : Constant  Value=PowerUnit_wb
  Wss : Outport  VectorParamsAs1DForOutWhenUnconnected=off
  wires:
  Sum/1 -> Wss/1  "Wss"
  wb(转速常参数)/1 -> Sum/2
  CR/1 -> Sum/1
  "throttle_cmd "/1 -> CR/1

== system test_p/四旋翼模型(简化)2/Kinetic model/Subsystem2 ==
  "throttle_cmd " : Inport
  CR : Gain  Gain=PowerUnit_CR
  Sum : Sum  Inputs=|++
  wb(转速常参数) : Constant  Value=PowerUnit_wb
  Wss : Outport  VectorParamsAs1DForOutWhenUnconnected=off
  wires:
  "throttle_cmd "/1 -> CR/1
  CR/1 -> Sum/1
  wb(转速常参数)/1 -> Sum/2
  Sum/1 -> Wss/1  "Wss"

== system test_p/四旋翼模型(简化)2/Kinetic model/Subsystem3 ==
  "throttle_cmd " : Inport
  CR : Gain  Gain=PowerUnit_CR
  Sum : Sum  Inputs=|++
  wb(转速常参数) : Constant  Value=PowerUnit_wb
  Wss : Outport  VectorParamsAs1DForOutWhenUnconnected=off
  wires:
  Sum/1 -> Wss/1  "Wss"
  wb(转速常参数)/1 -> Sum/2
  CR/1 -> Sum/1
  "throttle_cmd "/1 -> CR/1

== system test_p/四旋翼模型(简化)3/动力模型/Subsystem ==
  "throttle_cmd " : Inport
  CR : Gain  Gain=PowerUnit_CR
  Sum : Sum  Inputs=|++
  wb(转速常参数) : Constant  Value=PowerUnit_wb
  Wss : Outport  VectorParamsAs1DForOutWhenUnconnected=off
  wires:
  "throttle_cmd "/1 -> CR/1
  CR/1 -> Sum/1
  wb(转速常参数)/1 -> Sum/2
  Sum/1 -> Wss/1  "Wss"

== system test_p/四旋翼模型(简化)3/动力模型/Subsystem1 ==
  "throttle_cmd " : Inport
  CR : Gain  Gain=PowerUnit_CR
  Sum : Sum  Inputs=|++
  wb(转速常参数) : Constant  Value=PowerUnit_wb
  Wss : Outport  VectorParamsAs1DForOutWhenUnconnected=off
  wires:
  Sum/1 -> Wss/1  "Wss"
  wb(转速常参数)/1 -> Sum/2
  CR/1 -> Sum/1
  "throttle_cmd "/1 -> CR/1

== system test_p/四旋翼模型(简化)3/动力模型/Subsystem2 ==
  "throttle_cmd " : Inport
  CR : Gain  Gain=PowerUnit_CR
  Sum : Sum  Inputs=|++
  wb(转速常参数) : Constant  Value=PowerUnit_wb
  Wss : Outport  VectorParamsAs1DForOutWhenUnconnected=off
  wires:
  "throttle_cmd "/1 -> CR/1
  CR/1 -> Sum/1
  wb(转速常参数)/1 -> Sum/2
  Sum/1 -> Wss/1  "Wss"

== system test_p/四旋翼模型(简化)3/动力模型/Subsystem3 ==
  "throttle_cmd " : Inport
  CR : Gain  Gain=PowerUnit_CR
  Sum : Sum  Inputs=|++
  wb(转速常参数) : Constant  Value=PowerUnit_wb
  Wss : Outport  VectorParamsAs1DForOutWhenUnconnected=off
  wires:
  Sum/1 -> Wss/1  "Wss"
  wb(转速常参数)/1 -> Sum/2
  CR/1 -> Sum/1
  "throttle_cmd "/1 -> CR/1

== matlab function test_p/四旋翼模型(简化)1/姿态运动学/att_kine ==
  data: wbx input; roll_dot output; wby input; wbz input; pitch input; pitch_dot output; yaw_dot output; roll input
function [roll_dot,pitch_dot,yaw_dot] = att_kine(wbx,wby,wbz,pitch,roll)
%姿态运动学
roll_dot = wbx + tan(pitch)*sin(roll)*wby + tan(pitch)*cos(roll)*wbz;
pitch_dot = cos(roll)*wby - sin(roll)*wbz;
yaw_dot = (sin(roll)/cos(pitch))*wby + (cos(roll)/cos(pitch))*wbz;
end

== matlab function test_p/四旋翼模型(简化)1/控制效率模型/control_efficiency ==
  data: w1 input; f output; w2 input; w3 input; w4 input; t_x output; t_y output; t_z output; d input; ct input; cm input
function [f,t_x,t_y,t_z] = control_efficiency(w1,w2,w3,w4,d,ct,cm)
%控制效率模型
%X型机架
%3↓   1↑
%  \ /
%  / \
%2↑   4↓
%转速单位是弧度
f = -1*ct*(w1^2 + w2^2 + w3^2 + w4^2);%z轴朝下，所以拉力为负
t_x = d*ct*sin(pi/4)*(-w1^2 + w2^2 + w3^2 - w4^2) / 2;
t_y = d*ct*sin(pi/4)*(w1^2 - w2^2 + w3^2 - w4^2) / 2;
t_z = cm*(w1^2 + w2^2 - w3^2 - w4^2);
%十字型
% f = ct*(n1^2 + n2^2 + n3^2 + n4^2);
% tao_x = -d*ct*n2^2 + d*ct*n4^2;
% tao_y =  d*ct*n1^2 - d*ct*n3^2;
% tao_z = cm*(n1^2 - n2^2 + n3^2 - n4^2);
end

== matlab function test_p/动力电机分配2 ==
  data: thrust input; m1 output; m2 output; m3 output; m4 output; roll_pwm input; pitch_pwm input; yaw_pwm input
function [m1,m2,m3,m4] = motor_mixer(thrust,roll_pwm,pitch_pwm,yaw_pwm)
%输入的是都是占空比（0-1）之间
%输出在1000-2000
%这里采用x型机架，x型机架的分配和十字型的不一样


K = 1000;%将输入定在0-1000
pwm_base = 1000;%PWM从1000开始

m1 = (thrust - roll_pwm + pitch_pwm + yaw_pwm) * K + pwm_base;
m2 = (thrust + roll_pwm - pitch_pwm + yaw_pwm) * K + pwm_base;
m3 = (thrust + roll_pwm + pitch_pwm - yaw_pwm) * K + pwm_base;
m4 = (thrust - roll_pwm - pitch_pwm - yaw_pwm) * K + pwm_base;
end

== matlab function test_p/四旋翼模型(简化)2/Posture dynamics/att_dyna ==
  data: Ixx input; Iyy input; Izz input; t_x input; t_y input; t_z input; wbx_d output; wby_d output; wbz_d output
function [wbx_d,wby_d,wbz_d] = att_dyna(Ixx,Iyy,Izz,t_x,t_y,t_z)
% wb = [wbx wby wbz]';
% wb_cha = [   0 -wbz   wby;
%            wbz    0  -wbx;
%           -wby  wbx     0];
% I = [Ixx   0   0;
%        0 Iyy   0;
%        0   0 Izz];
I_inv = [1/Ixx     0     0;
             0 1/Iyy     0;
             0     0 1/Izz];
tao = [t_x t_y t_z]';
% G_x = Jrp * wby * (n1+n2-n3-n4);
% G_y = Jrp * wbx * (-n1-n2+n3+n4);
% G_z = 0;  
% G = [G_x G_y G_z]';
wb_dot = I_inv * (tao);
wbx_d = wb_dot(1,1);
wby_d = wb_dot(2,1);
wbz_d = wb_dot(3,1);
end

== matlab function test_p/四旋翼模型(简化)2/Posture Kinematics/att_kine ==
  data: wbx input; roll_dot output; wby input; wbz input; pitch input; pitch_dot output; yaw_dot output; roll input
function [roll_dot,pitch_dot,yaw_dot] = att_kine(wbx,wby,wbz,pitch,roll)
%姿态运动学
roll_dot = wbx + tan(pitch)*sin(roll)*wby + tan(pitch)*cos(roll)*wbz;
pitch_dot = cos(roll)*wby - sin(roll)*wbz;
yaw_dot = (sin(roll)/cos(pitch))*wby + (cos(roll)/cos(pitch))*wbz;
end

== matlab function test_p/四旋翼模型(简化)2/Control efficiency model/control_efficiency ==
  data: w1 input; f output; w2 input; w3 input; w4 input; t_x output; t_y output; t_z output; d input; ct input; cm input
function [f,t_x,t_y,t_z] = control_efficiency(w1,w2,w3,w4,d,ct,cm)
%控制效率模型
%X型机架
%3↓   1↑
%  \ /
%  / \
%2↑   4↓
%转速单位是弧度
f = -1*ct*(w1^2 + w2^2 + w3^2 + w4^2);%z轴朝下，所以拉力为负
t_x = d*ct*sin(pi/4)*(-w1^2 + w2^2 + w3^2 - w4^2) / 2;
t_y = d*ct*sin(pi/4)*(w1^2 - w2^2 + w3^2 - w4^2) / 2;
t_z = cm*(w1^2 + w2^2 - w3^2 - w4^2);
%十字型
% f = ct*(n1^2 + n2^2 + n3^2 + n4^2);
% tao_x = -d*ct*n2^2 + d*ct*n4^2;
% tao_y =  d*ct*n1^2 - d*ct*n3^2;
% tao_z = cm*(n1^2 - n2^2 + n3^2 - n4^2);
end

== matlab function test_p/动力电机分配3 ==
  data: thrust input; m1 output; m2 output; m3 output; m4 output; roll_pwm input; pitch_pwm input; yaw_pwm input
function [m1,m2,m3,m4] = motor_mixer(thrust,roll_pwm,pitch_pwm,yaw_pwm)
%输入的是都是占空比（0-1）之间
%输出在1000-2000
%这里采用x型机架，x型机架的分配和十字型的不一样


K = 1000;%将输入定在0-1000
pwm_base = 1000;%PWM从1000开始

m1 = (thrust - roll_pwm + pitch_pwm + yaw_pwm) * K + pwm_base;
m2 = (thrust + roll_pwm - pitch_pwm + yaw_pwm) * K + pwm_base;
m3 = (thrust + roll_pwm + pitch_pwm - yaw_pwm) * K + pwm_base;
m4 = (thrust - roll_pwm - pitch_pwm - yaw_pwm) * K + pwm_base;
end

== matlab function test_p/四旋翼模型(简化)3/姿态动力学/att_dyna ==
  data: Ixx input; Iyy input; Izz input; t_x input; t_y input; t_z input; wbx_d output; wby_d output; wbz_d output
function [wbx_d,wby_d,wbz_d] = att_dyna(Ixx,Iyy,Izz,t_x,t_y,t_z)
% wb = [wbx wby wbz]';
% wb_cha = [   0 -wbz   wby;
%            wbz    0  -wbx;
%           -wby  wbx     0];
% I = [Ixx   0   0;
%        0 Iyy   0;
%        0   0 Izz];
I_inv = [1/Ixx     0     0;
             0 1/Iyy     0;
             0     0 1/Izz];
tao = [t_x t_y t_z]';
% G_x = Jrp * wby * (n1+n2-n3-n4);
% G_y = Jrp * wbx * (-n1-n2+n3+n4);
% G_z = 0;  
% G = [G_x G_y G_z]';
wb_dot = I_inv * (tao);
wbx_d = wb_dot(1,1);
wby_d = wb_dot(2,1);
wbz_d = wb_dot(3,1);
end

== matlab function test_p/四旋翼模型(简化)3/姿态运动学/att_kine ==
  data: wbx input; roll_dot output; wby input; wbz input; pitch input; pitch_dot output; yaw_dot output; roll input
function [roll_dot,pitch_dot,yaw_dot] = att_kine(wbx,wby,wbz,pitch,roll)
%姿态运动学
roll_dot = wbx + tan(pitch)*sin(roll)*wby + tan(pitch)*cos(roll)*wbz;
pitch_dot = cos(roll)*wby - sin(roll)*wbz;
yaw_dot = (sin(roll)/cos(pitch))*wby + (cos(roll)/cos(pitch))*wbz;
end

== matlab function test_p/四旋翼模型(简化)/姿态动力学/att_dyna ==
  data: Ixx input; Iyy input; Izz input; t_x input; t_y input; t_z input; wbx_d output; wby_d output; wbz_d output
function [wbx_d,wby_d,wbz_d] = att_dyna(Ixx,Iyy,Izz,t_x,t_y,t_z)
% wb = [wbx wby wbz]';
% wb_cha = [   0 -wbz   wby;
%            wbz    0  -wbx;
%           -wby  wbx     0];
% I = [Ixx   0   0;
%        0 Iyy   0;
%        0   0 Izz];
I_inv = [1/Ixx     0     0;
             0 1/Iyy     0;
             0     0 1/Izz];
tao = [t_x t_y t_z]';
% G_x = Jrp * wby * (n1+n2-n3-n4);
% G_y = Jrp * wbx * (-n1-n2+n3+n4);
% G_z = 0;  
% G = [G_x G_y G_z]';
wb_dot = I_inv * (tao);
wbx_d = wb_dot(1,1);
wby_d = wb_dot(2,1);
wbz_d = wb_dot(3,1);
end

== matlab function test_p/四旋翼模型(简化)3/控制效率模型/control_efficiency ==
  data: w1 input; f output; w2 input; w3 input; w4 input; t_x output; t_y output; t_z output; d input; ct input; cm input
function [f,t_x,t_y,t_z] = control_efficiency(w1,w2,w3,w4,d,ct,cm)
%控制效率模型
%X型机架
%3↓   1↑
%  \ /
%  / \
%2↑   4↓
%转速单位是弧度
f = -1*ct*(w1^2 + w2^2 + w3^2 + w4^2);%z轴朝下，所以拉力为负
t_x = d*ct*sin(pi/4)*(-w1^2 + w2^2 + w3^2 - w4^2) / 2;
t_y = d*ct*sin(pi/4)*(w1^2 - w2^2 + w3^2 - w4^2) / 2;
t_z = cm*(w1^2 + w2^2 - w3^2 - w4^2);
%十字型
% f = ct*(n1^2 + n2^2 + n3^2 + n4^2);
% tao_x = -d*ct*n2^2 + d*ct*n4^2;
% tao_y =  d*ct*n1^2 - d*ct*n3^2;
% tao_z = cm*(n1^2 - n2^2 + n3^2 - n4^2);
end

== matlab function test_p/动力电机分配1 ==
  data: thrust input; m1 output; m2 output; m3 output; m4 output; roll_pwm input; pitch_pwm input; yaw_pwm input
function [m1,m2,m3,m4] = motor_mixer(thrust,roll_pwm,pitch_pwm,yaw_pwm)
%输入的是都是占空比（0-1）之间
%输出在1000-2000
%这里采用x型机架，x型机架的分配和十字型的不一样


K = 1000;%将输入定在0-1000
pwm_base = 1000;%PWM从1000开始

m1 = (thrust - roll_pwm + pitch_pwm + yaw_pwm) * K + pwm_base;
m2 = (thrust + roll_pwm - pitch_pwm + yaw_pwm) * K + pwm_base;
m3 = (thrust + roll_pwm + pitch_pwm - yaw_pwm) * K + pwm_base;
m4 = (thrust - roll_pwm - pitch_pwm - yaw_pwm) * K + pwm_base;
end

== matlab function test_p/四旋翼模型(简化)/姿态运动学/att_kine ==
  data: wbx input; roll_dot output; wby input; wbz input; pitch input; pitch_dot output; yaw_dot output; roll input
function [roll_dot,pitch_dot,yaw_dot] = att_kine(wbx,wby,wbz,pitch,roll)
%姿态运动学
roll_dot = wbx + tan(pitch)*sin(roll)*wby + tan(pitch)*cos(roll)*wbz;
pitch_dot = cos(roll)*wby - sin(roll)*wbz;
yaw_dot = (sin(roll)/cos(pitch))*wby + (cos(roll)/cos(pitch))*wbz;
end

== matlab function test_p/四旋翼模型(简化)/控制效率模型/control_efficiency ==
  data: w1 input; f output; w2 input; w3 input; w4 input; t_x output; t_y output; t_z output; d input; ct input; cm input
function [f,t_x,t_y,t_z] = control_efficiency(w1,w2,w3,w4,d,ct,cm)
%控制效率模型
%X型机架
%3↓   1↑
%  \ /
%  / \
%2↑   4↓
%转速单位是弧度
f = -1*ct*(w1^2 + w2^2 + w3^2 + w4^2);%z轴朝下，所以拉力为负
t_x = d*ct*sin(pi/4)*(-w1^2 + w2^2 + w3^2 - w4^2) / 2;
t_y = d*ct*sin(pi/4)*(w1^2 - w2^2 + w3^2 - w4^2) / 2;
t_z = cm*(w1^2 + w2^2 - w3^2 - w4^2);
%十字型
% f = ct*(n1^2 + n2^2 + n3^2 + n4^2);
% tao_x = -d*ct*n2^2 + d*ct*n4^2;
% tao_y =  d*ct*n1^2 - d*ct*n3^2;
% tao_z = cm*(n1^2 - n2^2 + n3^2 - n4^2);
end

== matlab function test_p/动力电机分配 ==
  data: thrust input; m1 output; m2 output; m3 output; m4 output; roll_pwm input; pitch_pwm input; yaw_pwm input
function [m1,m2,m3,m4] = motor_mixer(thrust,roll_pwm,pitch_pwm,yaw_pwm)
%输入的是都是占空比（0-1）之间
%输出在1000-2000
%这里采用x型机架，x型机架的分配和十字型的不一样


K = 1000;%将输入定在0-1000
pwm_base = 1000;%PWM从1000开始

m1 = (thrust - roll_pwm + pitch_pwm + yaw_pwm) * K + pwm_base;
m2 = (thrust + roll_pwm - pitch_pwm + yaw_pwm) * K + pwm_base;
m3 = (thrust + roll_pwm + pitch_pwm - yaw_pwm) * K + pwm_base;
m4 = (thrust - roll_pwm - pitch_pwm - yaw_pwm) * K + pwm_base;
end

== matlab function test_p/四旋翼模型(简化)1/姿态动力学/att_dyna ==
  data: Ixx input; Iyy input; Izz input; t_x input; t_y input; t_z input; wbx_d output; wby_d output; wbz_d output
function [wbx_d,wby_d,wbz_d] = att_dyna(Ixx,Iyy,Izz,t_x,t_y,t_z)
% wb = [wbx wby wbz]';
% wb_cha = [   0 -wbz   wby;
%            wbz    0  -wbx;
%           -wby  wbx     0];
% I = [Ixx   0   0;
%        0 Iyy   0;
%        0   0 Izz];
I_inv = [1/Ixx     0     0;
             0 1/Iyy     0;
             0     0 1/Izz];
tao = [t_x t_y t_z]';
% G_x = Jrp * wby * (n1+n2-n3-n4);
% G_y = Jrp * wbx * (-n1-n2+n3+n4);
% G_z = 0;  
% G = [G_x G_y G_z]';
wb_dot = I_inv * (tao);
wbx_d = wb_dot(1,1);
wby_d = wb_dot(2,1);
wbz_d = wb_dot(3,1);
end
